simulink model "FhHZirh3oA1jQvy1Xbs074Fj"  (R2017a)
settings: Solver=VariableStepAuto  StartTime=0.0  StopTime=0.001  RelTol=1e-3
libraries: commrandsrc3 x1, commdigbbndpm3 x1, dspsigops x1
settings Model: Creator=speychet  LastModifiedBy=speychet

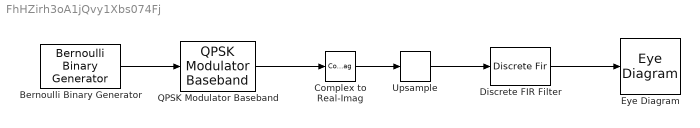
== system FhHZirh3oA1jQvy1Xbs074Fj ==
  Bernoulli Binary Generator : commrandsrc3/Bernoulli Binary Generator  ProbabilityOfZero=0.5  SeedSource=Auto  Seed=0  SampleTime=2e-7  SamplesPerFrame=2  OutputDataType=double  SimulateUsing=Interpreted execution
  Complex to Real-Imag : ComplexToRealImag  Output=Real
  Discrete FIR Filter : DiscreteFir  Coefficients=rcosdesign(0.4, 8, 4, 'normal')
  Eye Diagram : EyeDiagram
  QPSK Modulator Baseband : commdigbbndpm3/QPSK Modulator Baseband  InType=Bit  Enc=Gray  Ph=pi/4  outDtype=double  outWordLen=16  outUDDataType=sfix(16)  outFracLenMode=Best precision  outFracLen=15  outDataTypeStr=double  outLastDataTypeStr=double
  Upsample : dspsigops/Upsample  N=4  phase=0  RateOptions=Allow multirate processing  ic=0  mode=Unused parameter value
  wires:
  Discrete FIR Filter/1 -> Eye Diagram/1
  Complex to Real-Imag/1 -> Upsample/1
  Bernoulli Binary Generator/1 -> QPSK Modulator Baseband/1
  QPSK Modulator Baseband/1 -> Complex to Real-Imag/1
  Upsample/1 -> Discrete FIR Filter/1
